simulink model "mass_spring_damper"  (R2017a)
settings: Solver=VariableStepAuto  StartTime=0.0  StopTime=100  FixedStep=0.2  RelTol=1e-3
undefined symbols (not defined in the file or in its folder): b, k, m
settings Model: Creator=apuvvala  LastModifiedBy=apuvvala

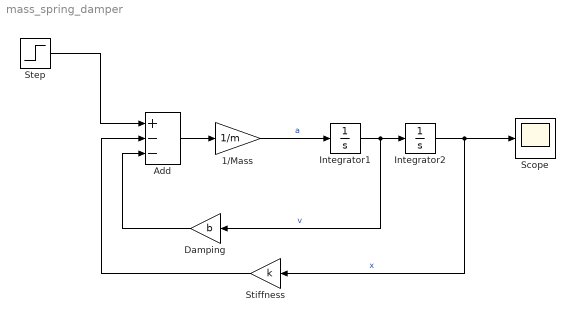
== system mass_spring_damper ==
  "1/Mass " : Gain  Gain=1/m  SaturateOnIntegerOverflow=on  OutDataTypeStr=Inherit: Same as input  ParamDataTypeStr=Inherit: Same as input
  Add : Sum  Inputs=+--
  Damping : Gain  Gain=b  SaturateOnIntegerOverflow=on  OutDataTypeStr=Inherit: Same as input  ParamDataTypeStr=Inherit: Same as input
  Integrator1 : Integrator
  Integrator2 : Integrator  InitialCondition=2
      settings: AttributesFormatString=x0 = %<InitialCondition> m
  Scope : Scope
  Step : Step  SampleTime=0
  Stiffness : Gain  Gain=k  SaturateOnIntegerOverflow=on  OutDataTypeStr=Inherit: Same as input  ParamDataTypeStr=Inherit: Same as input
  wires:
  "1/Mass "/1 -> Integrator1/1  "a"
  Integrator2/1 -> Scope/1, Stiffness/1  "x"
  Integrator1/1 -> Integrator2/1, Damping/1  "v"
  Add/1 -> "1/Mass "/1
  Step/1 -> Add/1
  Damping/1 -> Add/3
  Stiffness/1 -> Add/2
